simulink model "bess"  (R2024b)
settings: Solver=VariableStepAuto  StartTime=0.0  StopTime=10  RelTol=1e-3
undefined symbols (not defined in the file): Ion, Lithium
libraries: spsGroundLib x6, spsIdealSwitchLib x4, spsSeriesRLCBranchLib x3, spsThreePhaseSeriesRLCBranchLib x3, slpidlib x2, spsThreePhaseVIMeasurementLib x2, spsBatteryLib x1, spsBoostConverterLib x1, spsControlledVoltageSourceLib x1, spsCurrentMeasurementLib x1, eeDcVoltageController x1, spsPLL3phLib x1
settings Model: Creator=shanks  LastModifiedBy=shanks
settings SolverCC: ZeroCrossAlgorithm=Adaptive
settings DebuggingCC: AlgebraicLoopMsg=none  MaskedZcDiagnostic=none  IgnoredZcDiagnostic=none

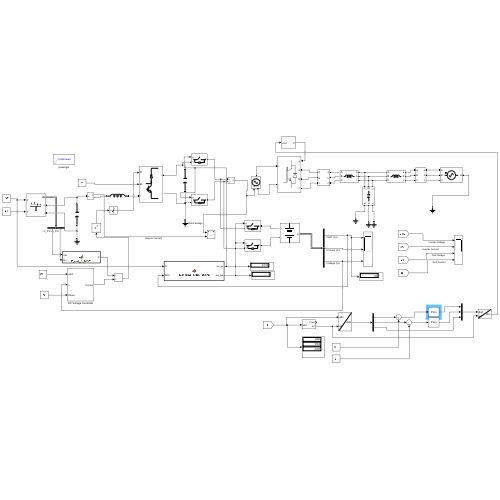
[thumbnail: Simulink's stored preview of the top-level diagram]
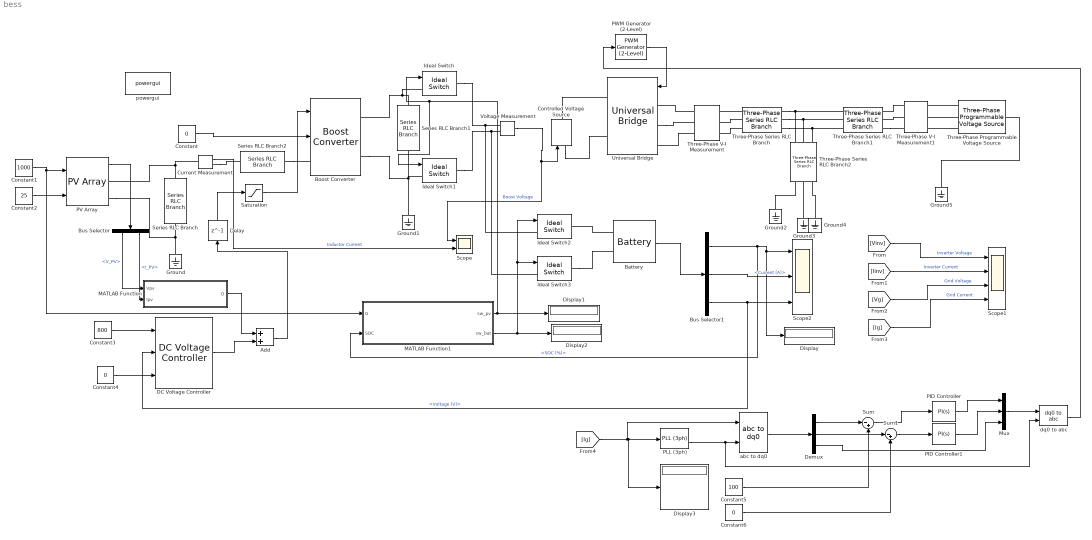
== system bess ==
  Add : Sum
  Battery : spsBatteryLib/Battery  BatType=Lithium-Ion  NomV=690  NomQ=54  SOC=100  Batt_Tr=30  PresetModel=on  MaxQ=54  MinV=517.5  FullV=803.1511  Dis_rate=23.4783  R=0.12778  Normal_OP=48.8348  expZone="[745.4662      2.653043]"
  Boost Converter : spsBoostConverterLib/Boost Converter  ModelType=Average model (D-controlled)  Ron=1e-3  Rs=1e6  Cs=inf  Vforward=[0,0]  Ron_Diode=1e-3  Rs_Diode=1e6  Cs_Diode=inf  Vf_Diode=1e-3  Rs_CurrentSource=inf  Ron_ACsource=1e-3
      settings: LibrarySourceBlock=sps_lib/Power Electronics/Boost Converter
  Bus Selector : BusSelector  OutputSignals=V_PV,I_PV
  Bus Selector1 : BusSelector  OutputSignals=SOC (%),Current (A),Voltage (V)
  Constant : Constant  Value=0
  Constant1 : Constant  Value=1000
  Constant2 : Constant  Value=25
  Constant3 : Constant  Value=800
  Constant4 : Constant  Value=0
  Constant5 : Constant  Value=100
  Constant6 : Constant  Value=0
  Controlled Voltage Source : spsControlledVoltageSourceLib/Controlled Voltage Source  Initialize=on  Source_Type=AC  Amplitude=0  Phase=0  Frequency=0  Measurements=None
  Current Measurement : spsCurrentMeasurementLib/Current Measurement  PhasorSimulation=off  OutputType=Complex  PSBequivalent=0
  DC Voltage Controller : eeDcVoltageController/DC Voltage Controller  Kp=1  Ki=0.5  Kaw=1  up=0.5  lo=0  Ts=-1  Tsd=0.001  Tf=0.001  ActZC=off  ActVdcFilter=on
      settings: LibrarySourceBlock=|
      | ee_sl_lib/General Machine
      | Control/DC Voltage Controller
  Delay : Delay  DelayLength=1
  Demux : Demux  Outputs=3
  Display{,1..3} (4 alike) : Display
  Ground{,1..5} (6 alike) : spsGroundLib/Ground  LConnTagsString=a
  Ideal Switch{,1..3} (4 alike) : spsIdealSwitchLib/Ideal Switch  Ron=0.001  Lon=0  IC=0  Rs=1e5  Cs=inf  Measurements=off
  MATLAB Function : MATLAB Function  TreatAsAtomicUnit=on
  MATLAB Function1 : MATLAB Function  TreatAsAtomicUnit=on
  Mux : Mux  Inputs=3
  PID Controller : slpidlib/PID Controller  Controller=PI  Form=Parallel  TimeDomain=Continuous-time  UseExternalTs=off  SampleTime=-1  IntegratorMethod=Forward Euler  FilterMethod=Forward Euler  ControllerParametersSource=internal  P=1e-6  I=1e-6  UseKiTs=off  D=0  UseExternalDerivativeSource=off  N=100  UseFilter=on  TunerSelectOption=Transfer Function Based (PID Tuner App)  InitialConditionSource=internal  InitialConditionForIntegrator=0  InitialConditionForFilter=0  DifferentiatorICPrevScaledInput=0  ExternalReset=none  TrackingMode=off  Kt=1  LimitOutput=off  SatLimitsSource=internal  UpperSaturationLimit=inf  LowerSaturationLimit=-inf  LinearizeAsGain=on  AntiWindupMode=none  Kb=1  LimitIntegrator=off  UpperIntegratorSaturationLimit=inf  LowerIntegratorSaturationLimit=-inf  POutMin=[]  POutMax=[]  IOutMin=[]  IOutMax=[]  DOutMin=[]  DOutMax=[]  NOutMin=[]  NOutMax=[]  SumOutMin=[]  SumOutMax=[]  SaturationOutMin=[]  SaturationOutMax=[]  PParamMin=[]  PParamMax=[]  IParamMin=[]  IParamMax=[]  DParamMin=[]  DParamMax=[]  NParamMin=[]  NParamMax=[]  KbParamMin=[]  KbParamMax=[]  KtParamMin=[]  KtParamMax=[]  KbOutMin=[]  KbOutMax=[]  KtOutMin=[]  KtOutMax=[]  IntegratorOutMin=[]  IntegratorOutMax=[]  FilterOutMin=[]  FilterOutMax=[]  SumI1OutMin=[]  SumI1OutMax=[]  SumI2OutMin=[]  SumI2OutMax=[]  SumI3OutMin=[]  SumI3OutMax=[]  SumI4OutMin=[]  SumI4OutMax=[]  SumDOutMin=[]  SumDOutMax=[]  DifferentiatorOutMin=[]  DifferentiatorOutMax=[]  FilterDiffOutCoefMin=[]  FilterDiffOutCoefMax=[]  ReciprocalOutMin=[]  ReciprocalOutMax=[]  SumDenOutMin=[]  SumDenOutMax=[]  SumNumOutMin=[]  SumNumOutMax=[]  DivideOutMin=[]  DivideOutMax=[]  UdiffTsProdOutMin=[]  UdiffTsProdOutMax=[]  NTsProdOutMin=[]  NTsProdOutMax=[]  UintegralTsProdOutMin=[]  UintegralTsProdOutMax=[]  UngainTsProdOutMin=[]  UngainTsProdOutMax=[]  ClampingZeroOutDataTypeStr=Inherit: Inherit via back propagation  ClampingZeroOutMin=[]  ClampingZeroOutMax=[]  FilterDenConstantOutDataTypeStr=Inherit: Inherit via back propagation  FilterDenConstantOutMin=[]  FilterDenConstantOutMax=[]  PCopyOutDataTypeStr=Inherit: Inherit via back propagation  PCopyOutMin=[]  PCopyOutMax=[]  NCopyOutDataTypeStr=Inherit: Inherit via back propagation  NCopyOutMin=[]  NCopyOutMax=[]  IntegratorContinuousStateAttributes=''  IntegratorStateMustResolveToSignalObject=off  IntegratorRTWStateStorageClass=Auto  FilterContinuousStateAttributes=''  FilterStateMustResolveToSignalObject=off  FilterRTWStateStorageClass=Auto  ParallelPVariant=InternalParameters  IdealPVariant=Disabled  IVariant=InternalParameters  DVariant=Disabled  IntegratorVariant=Continuous  SatVariant=Disabled  AWVariant=Passthrough  PCopyVariant=Disabled  TRVariant=Disabled  FdbkBlocksVariant=Forward  IdealPFdbkVariant=Disabled  SatFdbkVariant=Disabled  DerivativeFilterVariant=Disabled  NVariant=Disabled  NCopyVariant=Disabled_SignalSpec  FilterICVariant=Disabled  IntegratorICVariant=InternalICs  ExternalResetVariant=Disabled  TRSumVariant=Passthrough  SumFdbkVariant=Disabled  SumVariant=Sum_PI  TsampFilterVariant=InternalTs  TsampNgainVariant=Passthrough  TsampIntegralVariant=Disabled_SignalSpec  ExternalSaturationOutDataTypeStr=Inherit: Same as second input  DerivativeSourceVariant=Disabled  PreIntVariant=InternalPreInt
  PID Controller1 : slpidlib/PID Controller  Controller=PI  Form=Parallel  TimeDomain=Continuous-time  UseExternalTs=off  SampleTime=-1  IntegratorMethod=Forward Euler  FilterMethod=Forward Euler  ControllerParametersSource=internal  P=1e-6  I=1e-6  UseKiTs=off  D=0  UseExternalDerivativeSource=off  N=100  UseFilter=on  TunerSelectOption=Transfer Function Based (PID Tuner App)  InitialConditionSource=internal  InitialConditionForIntegrator=0  InitialConditionForFilter=0  DifferentiatorICPrevScaledInput=0  ExternalReset=none  TrackingMode=off  Kt=1  LimitOutput=off  SatLimitsSource=internal  UpperSaturationLimit=inf  LowerSaturationLimit=-inf  LinearizeAsGain=on  AntiWindupMode=none  Kb=1  LimitIntegrator=off  UpperIntegratorSaturationLimit=inf  LowerIntegratorSaturationLimit=-inf  POutMin=[]  POutMax=[]  IOutMin=[]  IOutMax=[]  DOutMin=[]  DOutMax=[]  NOutMin=[]  NOutMax=[]  SumOutMin=[]  SumOutMax=[]  SaturationOutMin=[]  SaturationOutMax=[]  PParamMin=[]  PParamMax=[]  IParamMin=[]  IParamMax=[]  DParamMin=[]  DParamMax=[]  NParamMin=[]  NParamMax=[]  KbParamMin=[]  KbParamMax=[]  KtParamMin=[]  KtParamMax=[]  KbOutMin=[]  KbOutMax=[]  KtOutMin=[]  KtOutMax=[]  IntegratorOutMin=[]  IntegratorOutMax=[]  FilterOutMin=[]  FilterOutMax=[]  SumI1OutMin=[]  SumI1OutMax=[]  SumI2OutMin=[]  SumI2OutMax=[]  SumI3OutMin=[]  SumI3OutMax=[]  SumI4OutMin=[]  SumI4OutMax=[]  SumDOutMin=[]  SumDOutMax=[]  DifferentiatorOutMin=[]  DifferentiatorOutMax=[]  FilterDiffOutCoefMin=[]  FilterDiffOutCoefMax=[]  ReciprocalOutMin=[]  ReciprocalOutMax=[]  SumDenOutMin=[]  SumDenOutMax=[]  SumNumOutMin=[]  SumNumOutMax=[]  DivideOutMin=[]  DivideOutMax=[]  UdiffTsProdOutMin=[]  UdiffTsProdOutMax=[]  NTsProdOutMin=[]  NTsProdOutMax=[]  UintegralTsProdOutMin=[]  UintegralTsProdOutMax=[]  UngainTsProdOutMin=[]  UngainTsProdOutMax=[]  ClampingZeroOutDataTypeStr=Inherit: Inherit via back propagation  ClampingZeroOutMin=[]  ClampingZeroOutMax=[]  FilterDenConstantOutDataTypeStr=Inherit: Inherit via back propagation  FilterDenConstantOutMin=[]  FilterDenConstantOutMax=[]  PCopyOutDataTypeStr=Inherit: Inherit via back propagation  PCopyOutMin=[]  PCopyOutMax=[]  NCopyOutDataTypeStr=Inherit: Inherit via back propagation  NCopyOutMin=[]  NCopyOutMax=[]  IntegratorContinuousStateAttributes=''  IntegratorStateMustResolveToSignalObject=off  IntegratorRTWStateStorageClass=Auto  FilterContinuousStateAttributes=''  FilterStateMustResolveToSignalObject=off  FilterRTWStateStorageClass=Auto  ParallelPVariant=InternalParameters  IdealPVariant=Disabled  IVariant=InternalParameters  DVariant=Disabled  IntegratorVariant=Continuous  SatVariant=Disabled  AWVariant=Passthrough  PCopyVariant=Disabled  TRVariant=Disabled  FdbkBlocksVariant=Forward  IdealPFdbkVariant=Disabled  SatFdbkVariant=Disabled  DerivativeFilterVariant=Disabled  NVariant=Disabled  NCopyVariant=Disabled_SignalSpec  FilterICVariant=Disabled  IntegratorICVariant=InternalICs  ExternalResetVariant=Disabled  TRSumVariant=Passthrough  SumFdbkVariant=Disabled  SumVariant=Sum_PI  TsampFilterVariant=InternalTs  TsampNgainVariant=Passthrough  TsampIntegralVariant=Disabled_SignalSpec  ExternalSaturationOutDataTypeStr=Inherit: Same as second input  DerivativeSourceVariant=Disabled  PreIntVariant=InternalPreInt
  PLL (3ph) : spsPLL3phLib/PLL (3ph)  Fmin=50  Par_Init=[0,50]  ParK=[180, 3200, 1]  TcD=1e-4  MaxRateChangeFreq=12  FilterCutOffFreq=25  Ts=0  AGC=on
  PV Array : spsPVArrayLib/PV Array  Npar=40  Nser=8  PlotType=array @ 1000 W/m2 & specified temperatures  S_vec="[ 1000  500  100 ]"  Temp_C_vec="[ 45 25  ]"  ModuleName=Ablytek 6PN6A225-A0  PlotWhenSelected=off  Pm=224.9856  Ncell=60  Voc=36.24  Isc=8.04  Vm=30.24  Im=7.44  beta_Voc_pc=-0.3624  alpha_Isc_pc=0.054801  beta_Voc=-0.13133  alpha_Isc=0.004406  IL=8.0514  I0=2.9114e-10  nI=0.97916  Rsh=136.1896  Rs=0.19316  RobustModel=off  RobustCellTemperature=313.3991  BAL=on  Tc=1e-6  Tfilter=5e-5
  PWM Generator (2-Level) : spsPWMGenerator2LevelLib/PWM Generator (2-Level)  ModulatorType=Three-phase bridge (6 pulses)  ModulatorMode=Unsynchronized  Fc=27*60  Pc=90  nF=27  MinMax="[ -1  1 ]"  SamplingTechnique=Natural  ModulatingSignals=off  m=1  Freq=50  Phase=0  Ts=0  ShowCarrierOutport=off
  Saturation : Saturate
  Scope : Scope  NumInputPorts=2
  Scope1 : Scope  NumInputPorts=4
  Scope2 : Scope  NumInputPorts=3
  Series RLC Branch : spsSeriesRLCBranchLib/Series RLC Branch  LConnTagsString=__new0  RConnTagsString=__new0  BranchType=C  Resistance=1  Inductance=1e-3  SetiL0=off  InitialCurrent=0  Capacitance=1e-6  Setx0=off  InitialVoltage=0  Measurements=None
  Series RLC Branch1 : spsSeriesRLCBranchLib/Series RLC Branch  LConnTagsString=__new0  RConnTagsString=__new0  BranchType=C  Resistance=1  Inductance=1e-3  SetiL0=off  InitialCurrent=0  Capacitance=1e-3  Setx0=off  InitialVoltage=0  Measurements=None
  Series RLC Branch2 : spsSeriesRLCBranchLib/Series RLC Branch  LConnTagsString=__new0  RConnTagsString=__new0  BranchType=L  Resistance=1  Inductance=1e-3  SetiL0=off  InitialCurrent=0  Capacitance=1e-6  Setx0=off  InitialVoltage=0  Measurements=None
  Sum : Sum  Inputs=|-+
  Sum1 : Sum  Inputs=|-+
  Three-Phase Programmable Voltage Source : spsThreePhaseProgrammableVoltageSourceLib/Three-Phase Programmable Voltage Source  PositiveSequence=[415 0 50]  VariationEntity=None  VariationType=Table of time-amplitude pairs  VariationTypeAlt=Step  VariationStep=0.5  VariationRate=10  VariationMagnitude=0.3  VariationFrequency=2  VariationTiming=[1 2]  VariationPhaseA=off  Amplitudes=[1 0.8 1.2 1.0]  TimeValues=[0 0.1 0.15 0.2]  HarmonicGeneration=off  HarmonicA=[3 0.2 -25 0]  HarmonicB=[2 0.15 35 2]  Timing="[0.05  3]"  BusType=swing  Pref=0  Qref=0  Qmin=-inf  Qmax=inf
  Three-Phase Series RLC Branch : spsThreePhaseSeriesRLCBranchLib/Three-Phase Series RLC Branch  LConnTagsString=A|B|C  RConnTagsString=A|B|C  BranchType=L  Resistance=1  Inductance=10e-3  Capacitance=1e-6  Measurements=None
  Three-Phase Series RLC Branch1 : spsThreePhaseSeriesRLCBranchLib/Three-Phase Series RLC Branch  LConnTagsString=A|B|C  RConnTagsString=A|B|C  BranchType=L  Resistance=1  Inductance=10e-3  Capacitance=1e-6  Measurements=None
  Three-Phase Series RLC Branch2 : spsThreePhaseSeriesRLCBranchLib/Three-Phase Series RLC Branch  LConnTagsString=A|B|C  RConnTagsString=A|B|C  BranchType=C  Resistance=1  Inductance=1e-3  Capacitance=100e-6  Measurements=None
  Three-Phase V-I Measurement : spsThreePhaseVIMeasurementLib/Three-Phase V-I Measurement  VoltageMeasurement=phase-to-ground  SetLabelV=on  LabelV=Vinv  Vpu=off  VpuLL=off  CurrentMeasurement=yes  SetLabelI=on  LabelI=Iinv  Ipu=off  Pbase=100e6  Vbase=500e3  OutputType=Complex  PhasorSimulation=off  PSBequivalent=0
  Three-Phase V-I Measurement1 : spsThreePhaseVIMeasurementLib/Three-Phase V-I Measurement  VoltageMeasurement=phase-to-ground  SetLabelV=on  LabelV=Vg  Vpu=off  VpuLL=off  CurrentMeasurement=yes  SetLabelI=on  LabelI=Ig  Ipu=off  Pbase=100e6  Vbase=500e3  OutputType=Complex  PhasorSimulation=off  PSBequivalent=0
  Universal Bridge : spsUniversalBridgeLib/Universal Bridge  Arms=3  SnubberResistance=1e5  SnubberCapacitance=inf  Device=IGBT / Diodes  Ron=1e-3  Lon=0  ForwardVoltages="[  0  0  ]"  ForwardVoltage=0  GTOparameters=[ 10e-6 , 20e-6 ]  IGBTparameters=[ 1e-6 , 2e-6 ]  Measurements=None  Measurements_2=None  converterType=Rectifier
  Voltage Measurement : spsVoltageMeasurementLib/Voltage Measurement  PhasorSimulation=off  OutputType=Complex  PSBequivalent=0
  abc to dq0 : spsabctodq0Lib/abc to dq0  Alignment=90 degrees behind phase A axis
  dq0 to abc : spsdq0toabcLib/dq0 to abc  Alignment=90 degrees behind phase A axis
  powergui : sps_lib/powergui  Priority=1  SimulationMode=Continuous  SampleTime=1e-6  frequency=60  Iterations=50  frequencyindice=0  Pbase=100e6  ErrMax=1e-4  UnitsV=kV  UnitsW=MW  buscounter=0  FunctionMessages=off  echomessages=off  EnableUseOfTLC=off  CurrentSourceSwitches=off  DisableSnubberDevices=off  DisableRonSwitches=off  DisableVfSwitches=off  DisplayEquations=off  AutomaticDiscreteSolvers=off  SolverType=Tustin/Backward Euler (TBE)  Interpol=off  ExternalGateDelay=off  methode=off  Ts=100  x0status=blocks  SPID=on  SwTol=0  HookPort=off  NonlinearTolerance=1e-4  nMaxIteration=100  ContinueOnMaxIteration=off  RestoreLinks=warning  ResistiveCurrentMeasurement=off  Frange=[0:2:500]  Ylog=off  Xlog=on  ShowGrid=off  save=off  variable=ZData  structure=0  ZoomFFT=off  StartTime=0.0  cycles=1  DisplayStyle=1  fundamental=60  FreqAxis=off  MaxFrequency=1000  frequencyindicesteady=1  RmsSteady=1  display=off
  wires:
  PV Array/1 -> Bus Selector/1
  Constant/1 -> Boost Converter/2
  Current Measurement/1 -> Scope/2  "Inductor Current"
  Voltage Measurement/1 -> Controlled Voltage Source/1, Scope/1  "Boost Voltage"
  Constant1/1 -> MATLAB Function1/1(G), PV Array/1
  Constant2/1 -> PV Array/2
  Bus Selector/1 -> MATLAB Function/1(Vpv)  "<V_PV>"
  Bus Selector/2 -> MATLAB Function/2(Ipv)  "<I_PV>"
  Delay/1 -> Saturation/1
  Saturation/1 -> Boost Converter/1
  PWM Generator (2-Level)/1 -> Universal Bridge/1
  [Vinv] -> Scope1/1  "Inverter Voltage"
  [Iinv] -> Scope1/2  "Inverter Current"
  [Vg] -> Scope1/3  "Grid Voltage"
  [Ig] -> Scope1/4  "Grid Current"
  Battery/1 -> Bus Selector1/1
  Bus Selector1/1 -> MATLAB Function1/2(SOC), Display/1, Scope2/1  "<SOC (%)>"
  Bus Selector1/2 -> Scope2/2  "<Current (A)>"
  Bus Selector1/3 -> DC Voltage Controller/2, Scope2/3  "<Voltage (V)>"
  MATLAB Function1/1(sw_pv) -> Display1/1, Ideal Switch1/1, Ideal Switch/1
  MATLAB Function1/2(sw_bat) -> Display2/1, Ideal Switch3/1, Ideal Switch2/1
  Constant3/1 -> DC Voltage Controller/1
  Constant4/1 -> DC Voltage Controller/3
  MATLAB Function/1(D) -> Add/1
  DC Voltage Controller/1 -> Add/2
  Add/1 -> Delay/1
  [Ig] -> abc to dq0/1, Display3/1, PLL (3ph)/1
  PLL (3ph)/2 -> dq0 to abc/2, abc to dq0/2
  abc to dq0/1 -> Demux/1
  Demux/1 -> Sum/1
  Constant5/1 -> Sum/2
  Demux/2 -> Sum1/1
  Constant6/1 -> Sum1/2
  Sum/1 -> PID Controller/1
  Sum1/1 -> PID Controller1/1
  Mux/1 -> dq0 to abc/1
  PID Controller/1 -> Mux/1
  PID Controller1/1 -> Mux/2
  Demux/3 -> Mux/3
  dq0 to abc/1 -> PWM Generator (2-Level)/1
  connections:
  Series RLC Branch/LConn1 -- Current Measurement/LConn1 -- PV Array/RConn1
  PV Array/RConn2 -- Ground/LConn1 -- Series RLC Branch/RConn1
  Series RLC Branch1/LConn1 -- Boost Converter/RConn1 -- Ideal Switch/LConn1
  Boost Converter/RConn2 -- Ground1/LConn1 -- Ideal Switch1/LConn1 -- Series RLC Branch1/RConn1
  Series RLC Branch2/LConn1 -- Boost Converter/LConn1
  Current Measurement/RConn1 -- Series RLC Branch2/RConn1
  Controlled Voltage Source/RConn1 -- Universal Bridge/RConn1
  Controlled Voltage Source/LConn1 -- Universal Bridge/RConn2
  Three-Phase Series RLC Branch/RConn1 -- Three-Phase Series RLC Branch1/LConn1 -- Three-Phase Series RLC Branch2/LConn1
  Three-Phase Series RLC Branch/RConn2 -- Three-Phase Series RLC Branch1/LConn2 -- Three-Phase Series RLC Branch2/LConn2
  Three-Phase Series RLC Branch/RConn3 -- Three-Phase Series RLC Branch1/LConn3 -- Three-Phase Series RLC Branch2/LConn3
  Ground2/LConn1 -- Three-Phase Series RLC Branch2/RConn1
  Ground3/LConn1 -- Three-Phase Series RLC Branch2/RConn2
  Ground4/LConn1 -- Three-Phase Series RLC Branch2/RConn3
  Three-Phase V-I Measurement/LConn1 -- Universal Bridge/LConn1
  Universal Bridge/LConn2 -- Three-Phase V-I Measurement/LConn2
  Three-Phase V-I Measurement/LConn3 -- Universal Bridge/LConn3
  Three-Phase Series RLC Branch/LConn1 -- Three-Phase V-I Measurement/RConn1
  Three-Phase Series RLC Branch/LConn2 -- Three-Phase V-I Measurement/RConn2
  Three-Phase Series RLC Branch/LConn3 -- Three-Phase V-I Measurement/RConn3
  Three-Phase V-I Measurement1/LConn1 -- Three-Phase Series RLC Branch1/RConn1
  Three-Phase V-I Measurement1/LConn2 -- Three-Phase Series RLC Branch1/RConn2
  Three-Phase Series RLC Branch1/RConn3 -- Three-Phase V-I Measurement1/LConn3
  Three-Phase Programmable Voltage Source/RConn1 -- Three-Phase V-I Measurement1/RConn1
  Three-Phase Programmable Voltage Source/RConn2 -- Three-Phase V-I Measurement1/RConn2
  Three-Phase Programmable Voltage Source/RConn3 -- Three-Phase V-I Measurement1/RConn3
  Ground5/LConn1 -- Three-Phase Programmable Voltage Source/LConn1
  Ideal Switch/RConn1 -- Ideal Switch2/LConn1 -- Voltage Measurement/LConn1
  Ideal Switch1/RConn1 -- Ideal Switch3/LConn1 -- Voltage Measurement/LConn2
  Battery/LConn1 -- Ideal Switch2/RConn1
  Ideal Switch3/RConn1 -- Battery/LConn2

== matlab function bess/MATLAB Function ==
  settings: updateMethod=DISCRETE
  data: Vpv input; D output; Ipv input
function D = P_and_O_MPPT(Vpv, Ipv)

% Perturb and Observe MPPT Algorithm
% Inputs:
% Vpv = PV voltage
% Ipv = PV current
%
% Output:
% D = duty cycle for boost converter

persistent Vprev Pprev Dprev

% Initial values
if isempty(Vprev)
    Vprev = 0;
    Pprev = 0;
    Dprev = 0.5;   % initial duty cycle
end

% Step size for perturbation
deltaD = 0.001;

% Duty cycle limits
Dmax = 0.9;
Dmin = 0.1;

% Present PV power
Ppv = Vpv * Ipv;

% Change in voltage and power
dV = Vpv - Vprev;
dP = Ppv - Pprev;

% P&O logic
if dP > 0
    if dV > 0
        D = Dprev - deltaD;
    else
        D = Dprev + deltaD;
    end
else
    if dV > 0
        D = Dprev + deltaD;
    else
        D = Dprev - deltaD;
    end
end

% Limit duty cycle
if D > Dmax
    D = Dmax;
elseif D < Dmin
    D = Dmin;
end

% Store previous values
Vprev = Vpv;
Pprev = Ppv;
Dprev = D;

end

== matlab function bess/MATLAB Function1 ==
  settings: updateMethod=DISCRETE
  data: G input; sw_pv output; SOC input; sw_bat output
function [sw_pv, sw_bat] = dual_ramp_switch_control(G, SOC)

% G   = irradiance in W/m^2
% SOC = battery state of charge in %

persistent pv_ref bat_ref pv_ramp bat_ramp

if isempty(pv_ref)
    pv_ref = 0;
    bat_ref = 0;
    pv_ramp = 0;
    bat_ramp = 0;
end

% -------------------------------
% Switching logic
% -------------------------------

if G > 700
    % Daytime condition
    pv_ref = 1;      % boost converter to inverter ON
    bat_ref = 0;     % battery switch OFF

elseif G < 300 && SOC > 80
    % Night/low irradiance and battery sufficiently charged
    pv_ref = 0;      % boost converter to inverter OFF
    bat_ref = 1;     % battery switch ON

elseif G < 300 && SOC <= 80
    % Low irradiance but battery not sufficiently charged
    pv_ref = 0;
    bat_ref = 0;

else
    % Between 300 and 700 W/m^2, hold previous state
    pv_ref = pv_ref;
    bat_ref = bat_ref;
end

% -------------------------------
% Ramp parameters
% -------------------------------

Ts = 1e-6;           % 1 us sampling time
ramp_time = 0.05;    % 50 ms ramp time

step = Ts / ramp_time;

% -------------------------------
% PV switch ramp
% -------------------------------

if pv_ramp < pv_ref
    pv_ramp = pv_ramp + step;
    if pv_ramp > pv_ref
        pv_ramp = pv_ref;
    end
elseif pv_ramp > pv_ref
    pv_ramp = pv_ramp - step;
    if pv_ramp < pv_ref
        pv_ramp = pv_ref;
    end
end

% -------------------------------
% Battery switch ramp
% -------------------------------

if bat_ramp < bat_ref
    bat_ramp = bat_ramp + step;
    if bat_ramp > bat_ref
        bat_ramp = bat_ref;
    end
elseif bat_ramp > bat_ref
    bat_ramp = bat_ramp - step;
    if bat_ramp < bat_ref
        bat_ramp = bat_ref;
    end
end

sw_pv = pv_ramp;
sw_bat = bat_ramp;

end
